simulink model "NoVCU"  (R2026b)
undefined symbols (not defined in the file): PlntEngTqMax
settings Model: Creator=The MathWorks, Inc.  LastModifiedBy=The MathWorks, Inc.

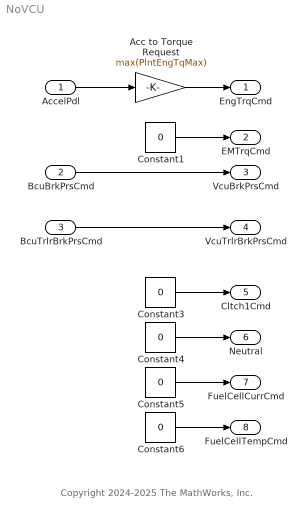
== system NoVCU ==
  note: Copyright 2024-2025 The MathWorks, Inc.
  AccelPdl : Inport
  BcuBrkPrsCmd : Inport  Port=2
  BcuTrlrBrkPrsCmd : Inport  Port=3
  Acc to Torque Request : Gain  Gain=max(PlntEngTqMax)
  Constant{1,3..6} (5 alike) : Constant  Value=0  SampleTime=-1
  EngTrqCmd : Outport  OutDataTypeStr=double  PortDimensions=1  VectorParamsAs1DForOutWhenUnconnected=off
  EMTrqCmd : Outport  Port=2  VectorParamsAs1DForOutWhenUnconnected=off
  VcuBrkPrsCmd : Outport  Port=3  PortDimensions=4  VectorParamsAs1DForOutWhenUnconnected=off
  VcuTrlrBrkPrsCmd : Outport  Port=4  PortDimensions=6  VectorParamsAs1DForOutWhenUnconnected=off
  Cltch1Cmd : Outport  Port=5  PortDimensions=1  VectorParamsAs1DForOutWhenUnconnected=off
  Neutral : Outport  Port=6  PortDimensions=1  VectorParamsAs1DForOutWhenUnconnected=off
  FuelCellCurrCmd : Outport  Port=7
  FuelCellTempCmd : Outport  Port=8
  wires:
  BcuTrlrBrkPrsCmd/1 -> VcuTrlrBrkPrsCmd/1
  Constant1/1 -> EMTrqCmd/1
  Constant3/1 -> Cltch1Cmd/1
  AccelPdl/1 -> Acc to Torque Request/1
  Constant5/1 -> FuelCellCurrCmd/1
  Acc to Torque Request/1 -> EngTrqCmd/1
  BcuBrkPrsCmd/1 -> VcuBrkPrsCmd/1
  Constant4/1 -> Neutral/1
  Constant6/1 -> FuelCellTempCmd/1
